simulink model "PMSM_FOC_DualPlant_ClosedLoop_v21"  (R2024a)
settings: Solver=FixedStepDiscrete  StartTime=0.0  StopTime=2.0  FixedStep=0.0001  RelTol=1e-3
model workspace (MAT data in the model file):
  FOC_Native_CurrentIntegratorLimit = Simulink.Parameter
  FOC_Native_CurrentIntegratorLimit.Value = 30
  FOC_Native_CurrentIntegratorLimit.Complexity = 'real'
  FOC_Native_CurrentIntegratorLimit.Dimensions = [1 1]
  FOC_Native_CurrentIntegratorLimit.DataType = 'single'
  FOC_Native_CurrentPeriod = Simulink.Parameter
  FOC_Native_CurrentPeriod.Value = 9.99999974738e-05
  FOC_Native_CurrentPeriod.Complexity = 'real'
  FOC_Native_CurrentPeriod.Dimensions = [1 1]
  FOC_Native_CurrentPeriod.DataType = 'single'
  FOC_Native_DutyMax = Simulink.Parameter
  FOC_Native_DutyMax.Value = 0.980000019073
  FOC_Native_DutyMax.Complexity = 'real'
  FOC_Native_DutyMax.Dimensions = [1 1]
  FOC_Native_DutyMax.DataType = 'single'
  FOC_Native_DutyMin = Simulink.Parameter
  FOC_Native_DutyMin.Value = 0.019999999553
  FOC_Native_DutyMin.Complexity = 'real'
  FOC_Native_DutyMin.Dimensions = [1 1]
  FOC_Native_DutyMin.DataType = 'single'
  FOC_Native_FluxPM = Simulink.Parameter
  FOC_Native_FluxPM.Value = 0.0500000007451
  FOC_Native_FluxPM.Complexity = 'real'
  FOC_Native_FluxPM.Dimensions = [1 1]
  FOC_Native_FluxPM.DataType = 'single'
  FOC_Native_IqLimit = Simulink.Parameter
  FOC_Native_IqLimit.Value = 8
  FOC_Native_IqLimit.Complexity = 'real'
  FOC_Native_IqLimit.Dimensions = [1 1]
  FOC_Native_IqLimit.DataType = 'single'
  FOC_Native_KiCurrent = Simulink.Parameter
  FOC_Native_KiCurrent.Value = 500
  FOC_Native_KiCurrent.Complexity = 'real'
  FOC_Native_KiCurrent.Dimensions = [1 1]
  FOC_Native_KiCurrent.DataType = 'single'
  FOC_Native_KiSpeed = Simulink.Parameter
  FOC_Native_KiSpeed.Value = 0.0500000007451
  FOC_Native_KiSpeed.Complexity = 'real'
  FOC_Native_KiSpeed.Dimensions = [1 1]
  FOC_Native_KiSpeed.DataType = 'single'
  FOC_Native_KpCurrent = Simulink.Parameter
  FOC_Native_KpCurrent.Value = 1
  FOC_Native_KpCurrent.Complexity = 'real'
  FOC_Native_KpCurrent.Dimensions = [1 1]
  FOC_Native_KpCurrent.DataType = 'single'
  FOC_Native_KpSpeed = Simulink.Parameter
  FOC_Native_KpSpeed.Value = 0.019999999553
  FOC_Native_KpSpeed.Complexity = 'real'
  FOC_Native_KpSpeed.Dimensions = [1 1]
  FOC_Native_KpSpeed.DataType = 'single'
  FOC_Native_Ld = Simulink.Parameter
  FOC_Native_Ld.Value = 0.0010000000475
  FOC_Native_Ld.Complexity = 'real'
  FOC_Native_Ld.Dimensions = [1 1]
  FOC_Native_Ld.DataType = 'single'
  FOC_Native_Lq = Simulink.Parameter
  FOC_Native_Lq.Value = 0.0010000000475
  FOC_Native_Lq.Complexity = 'real'
  FOC_Native_Lq.Dimensions = [1 1]
  FOC_Native_Lq.DataType = 'single'
  FOC_Native_PolePairs = Simulink.Parameter
  FOC_Native_PolePairs.Value = 4
  FOC_Native_PolePairs.Complexity = 'real'
  FOC_Native_PolePairs.Dimensions = [1 1]
  FOC_Native_PolePairs.DataType = 'single'
  FOC_Native_SpeedPeriod = Simulink.Parameter
  FOC_Native_SpeedPeriod.Value = 0.0010000000475
  FOC_Native_SpeedPeriod.Complexity = 'real'
  FOC_Native_SpeedPeriod.Dimensions = [1 1]
  FOC_Native_SpeedPeriod.DataType = 'single'
  FOC_Native_VoltageLimit = Simulink.Parameter
  FOC_Native_VoltageLimit.Value = 26
  FOC_Native_VoltageLimit.Complexity = 'real'
  FOC_Native_VoltageLimit.Dimensions = [1 1]
  FOC_Native_VoltageLimit.DataType = 'single'
  NATIVE_INV_SQRT3 = 0.577350258827
  NATIVE_RAD_S_TO_RPM = 9.54929637909
  NATIVE_RPM_TO_RAD_S = 0.104719758034
  NATIVE_SQRT3_BY2 = 0.866025388241
  PMSM_Native_B = 9.99999974738e-05
  PMSM_Native_J = 0.00200000009499
  PMSM_Native_Rs = 0.40000000596
  PMSM_PLANT_SELECTION = 2
values from neighbouring files (symbols this model uses):
  FOC_Native_CurrentIntegratorLimit = 30.0    [PMSM_FOC_Data.sldd]
  FOC_Native_CurrentPeriod = 0.0001    [PMSM_FOC_Data.sldd]
  FOC_Native_DutyMax = 0.98    [PMSM_FOC_Data.sldd]
  FOC_Native_DutyMin = 0.02    [PMSM_FOC_Data.sldd]
  FOC_Native_FluxPM = 0.05    [PMSM_FOC_Data.sldd]
  FOC_Native_IqLimit = 8.0    [PMSM_FOC_Data.sldd]
  FOC_Native_KiCurrent = 500.0    [PMSM_FOC_Data.sldd]
  FOC_Native_KiSpeed = 0.05    [PMSM_FOC_Data.sldd]
  FOC_Native_KpCurrent = 1.0    [PMSM_FOC_Data.sldd]
  FOC_Native_KpSpeed = 0.02    [PMSM_FOC_Data.sldd]
  FOC_Native_Ld = 0.001    [PMSM_FOC_Data.sldd]
  FOC_Native_Lq = 0.001    [PMSM_FOC_Data.sldd]
  FOC_Native_PolePairs = 4.0    [PMSM_FOC_Data.sldd]
  FOC_Native_SpeedPeriod = 0.001    [PMSM_FOC_Data.sldd]
  FOC_Native_VoltageLimit = 26.0    [PMSM_FOC_Data.sldd]
libraries: mcbhdlplantlib x2
settings Model: Creator=18283  LastModifiedBy=18283
settings DataIOCC: SignalLogging=off

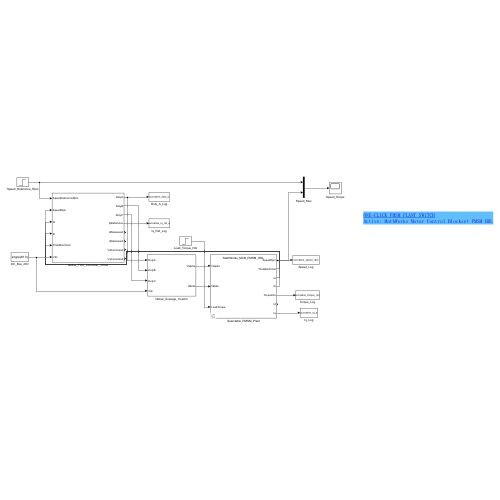
[thumbnail: Simulink's stored preview of the top-level diagram]
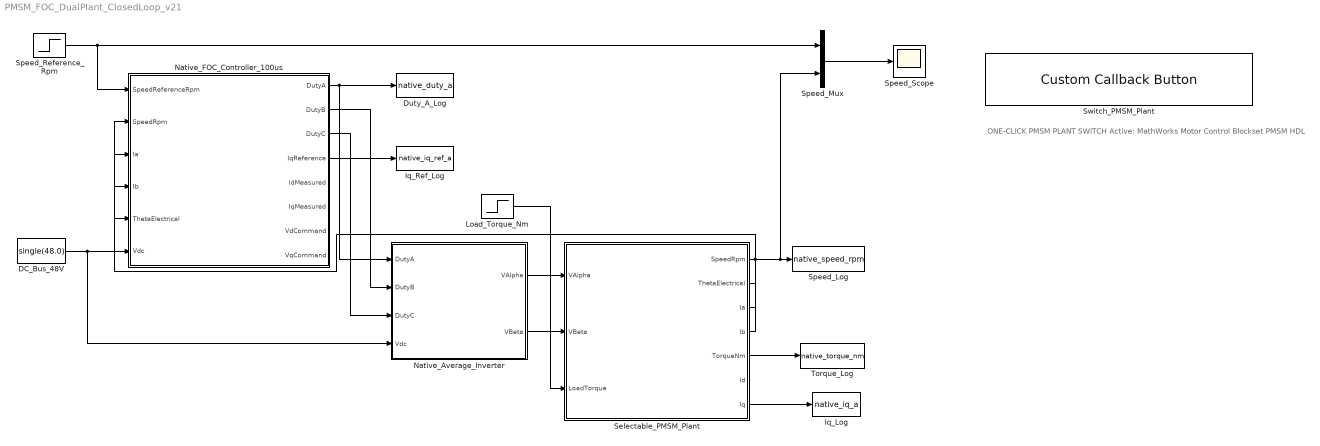
== system PMSM_FOC_DualPlant_ClosedLoop_v21 ==
  note: ONE-CLICK PMSM PLANT SWITCH
      | Active: MathWorks Motor Control Blockset PMSM HDL
  DC_Bus_48V : Constant  Value=single(48.0)  OutDataTypeStr=single
  Duty_A_Log : ToWorkspace  VariableName=native_duty_a  SaveFormat=Timeseries  SampleTime=-1
      settings: MaxDataPoints=20000
  Iq_Log : ToWorkspace  VariableName=native_iq_a  SaveFormat=Timeseries  SampleTime=-1
      settings: MaxDataPoints=20000
  Iq_Ref_Log : ToWorkspace  VariableName=native_iq_ref_a  SaveFormat=Timeseries  SampleTime=-1
      settings: MaxDataPoints=20000
  Load_Torque_Nm : Step  Time=0.5  After=0.2  OutDataTypeStr=single  SampleTime=0.0001
  Native_Average_Inverter : Subsystem
  Native_FOC_Controller_100us : Subsystem
  Selectable_PMSM_Plant : Subsystem  Variant=on  VariantControl=Native_Discrete_PMSM_Plant
  Speed_Log : ToWorkspace  VariableName=native_speed_rpm  SaveFormat=Timeseries  SampleTime=-1
      settings: MaxDataPoints=20000
  Speed_Mux : Mux  Inputs=2
  Speed_Reference_Rpm : Step  Time=0.05  After=1000  OutDataTypeStr=single  SampleTime=0.0001
  Speed_Scope : Scope
  Switch_PMSM_Plant : CustomCallbackButton  Configuration="{\"components\":[{\"name\":\"BackgroundImageComponent\",\"settings\":{\"image\":{\"size\":[0,0],\"src\":\"default\",\"srcOrientation\":\"Right\"},\"position\":[0,0,1,1]}},{\"name\":\"ButtonStateComponent\",\"settings\":{\"buttonType\":\"momentary\",\"clickFcn\":\"run(fullfile('G:\\\\Data\\\\GitFiles\\\\MatlabProgram\\\\Matlab_Projects\\\\PMSM_FOC\\\\model_codegen\\\\PMSM_FOC_DualPlant_v2.1.0','switch_pmsm_plant_v21.m'))\",\"onValue\":1,\"position\":[0,0,1,1],\"pressDelay\":\"500\",\"pressFcn\":\"\",\"repeatInterval\":\"0\",\"states\":[{\"horizontalAlignment\":\"center\",\"image\":{\"position\":[0,0,1,1],\"src\":\"default\",\"srcOrientation\":\"Right\"},\"label\":{\"color\":[0.01176470588,0.01176470588,0.01176470588,1],\"icon\":{\"size\":[0,0],\"src\":\"default\",\"srcOrientation\":\"Right\"},\"iconPlacement\":\"left\",\"text\":{\"content\":\"Active: MathWorks MCB PMSM HDL (click to switch)\"}},\"labelOffset\":[0,0],\"verticalAlignment\":\"middle\"},{\"horizontalAlignment\":\"center\",\"image\":{\"position\":[0,0,1,1],\"src\":\"default\",\"srcOrientation\":\"Right\"},\"label\":{\"color\":[0.01176470588,0.01176470588,0.01176470588,1],\"icon\":{\"size\":[0,0],\"src\":\"default\",\"srcOrientation\":\"Right\"},\"iconPlacement\":\"left\",\"text\":{\"content\":\"Active: MathWorks MCB PMSM HDL (click to switch)\"}},\"labelOffset\":[0,0],\"verticalAlignment\":\"middle\"},{\"horizontalAlignment\":\"center\",\"image\":{\"position\":[0,0,1,1],\"src\":\"default\",\"srcOrientation\":\"Right\"},\"label\":{\"color\":[0.01176470588,0.01176470588,0.01176470588,1],\"icon\":{\"size\":[0,0],\"src\":\"default\",\"srcOrientation\":\"Right\"},\"iconPlacement\":\"left\",\"text\":{\"content\":\"Active: MathWorks MCB PMSM HDL (click to switch)\"}},\"labelOffset\":[0,0],\"verticalAlignment\":\"middle\"},{\"horizontalAlignment\":\"center\",\"image\":{\"position\":[0,0,1,1],\"src\":\"default\",\"srcOrientation\":\"Right\"},\"label\":{\"color\":[0.01176470588,0.01176470588,0.01176470588,1],\"icon\":{\"size\":[0,0],\"src\":\"default\",\"srcOrientation\":\"Right\"},\"iconPlacement\":\"left\",\"text\":{\"content\":\"Active: MathWorks MCB PMSM HDL (click to switch)\"}},\"labelOffset\":[0,0],\"verticalAlignment\":\"middle\"}]}},{\"name\":\"ForegroundImageComponent\",\"settings\":{\"image\":{\"size\":[0,0],\"src\":\"default\",\"srcOrientation\":\"Right\"},\"isForeground\":1,\"position\":[0,0,1,1]}}],\"settings\":{\"BindingType\":\"standalone\",\"backgroundColor\":[244,244,244,1],\"backgroundOffset\":0.2,\"backgroundOpacity\":1,\"fixedAspectRatio\":\"off\",\"foregroundColor\":[0.01176470588,0.01176470588,0.01176470588,1],\"migratedFromLegacy\":true,\"useBackgroundColor\":true,\"variant\":\"callback\",\"version\":\"R2023a\"},\"type\":\"Button\"}"  CustomBackgroundColor="{\"color\":[0.9568627451,0.9568627451,0.9568627451],\"show\":true}"
  Torque_Log : ToWorkspace  VariableName=native_torque_nm  SaveFormat=Timeseries  SampleTime=-1
      settings: MaxDataPoints=20000
  wires:
  Native_FOC_Controller_100us/1(DutyA) -> Native_Average_Inverter/1(DutyA), Duty_A_Log/1
  Speed_Reference_Rpm/1 -> Speed_Mux/1, Native_FOC_Controller_100us/1(SpeedReferenceRpm)
  DC_Bus_48V/1 -> Native_Average_Inverter/4(Vdc), Native_FOC_Controller_100us/6(Vdc)
  Native_FOC_Controller_100us/2(DutyB) -> Native_Average_Inverter/2(DutyB)
  Native_FOC_Controller_100us/3(DutyC) -> Native_Average_Inverter/3(DutyC)
  Native_FOC_Controller_100us/4(IqReference) -> Iq_Ref_Log/1
  Speed_Mux/1 -> Speed_Scope/1
  Native_Average_Inverter/1(VAlpha) -> Selectable_PMSM_Plant/1(VAlpha)
  Native_Average_Inverter/2(VBeta) -> Selectable_PMSM_Plant/2(VBeta)
  Load_Torque_Nm/1 -> Selectable_PMSM_Plant/3(LoadTorque)
  Selectable_PMSM_Plant/1(SpeedRpm) -> Speed_Mux/2, Speed_Log/1, Native_FOC_Controller_100us/2(SpeedRpm)
  Selectable_PMSM_Plant/2(ThetaElectrical) -> Native_FOC_Controller_100us/5(ThetaElectrical)
  Selectable_PMSM_Plant/3(Ia) -> Native_FOC_Controller_100us/3(Ia)
  Selectable_PMSM_Plant/4(Ib) -> Native_FOC_Controller_100us/4(Ib)
  Selectable_PMSM_Plant/5(TorqueNm) -> Torque_Log/1
  Selectable_PMSM_Plant/7(Iq) -> Iq_Log/1

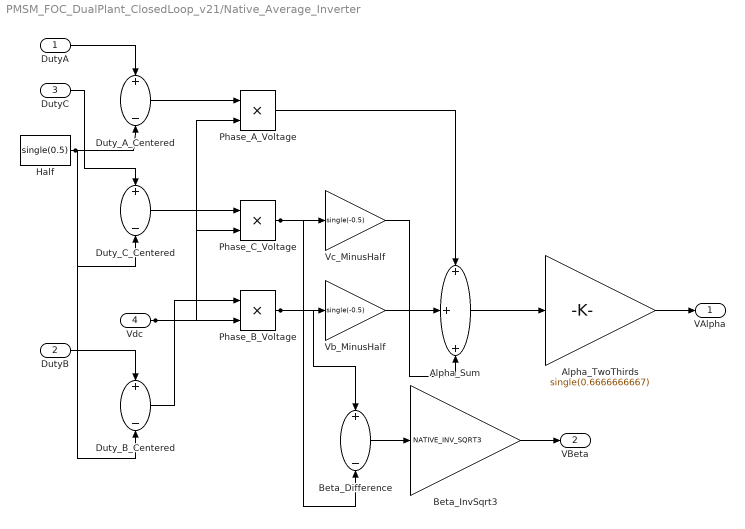
== system PMSM_FOC_DualPlant_ClosedLoop_v21/Native_Average_Inverter ==
  DutyA : Inport  OutDataTypeStr=single
  DutyB : Inport  Port=2  OutDataTypeStr=single
  DutyC : Inport  Port=3  OutDataTypeStr=single
  Vdc : Inport  Port=4  OutDataTypeStr=single
  Alpha_Sum : Sum  Inputs=+++
  Alpha_TwoThirds : Gain  Gain=single(0.6666666667)
  Beta_Difference : Sum  Inputs=+-
  Beta_InvSqrt3 : Gain  Gain=NATIVE_INV_SQRT3
  Duty_A_Centered : Sum  Inputs=+-
  Duty_B_Centered : Sum  Inputs=+-
  Duty_C_Centered : Sum  Inputs=+-
  Half : Constant  Value=single(0.5)  OutDataTypeStr=single
  Phase_A_Voltage : Product  Inputs=**
  Phase_B_Voltage : Product  Inputs=**
  Phase_C_Voltage : Product  Inputs=**
  Vb_MinusHalf : Gain  Gain=single(-0.5)
  Vc_MinusHalf : Gain  Gain=single(-0.5)
  VAlpha : Outport  OutDataTypeStr=single
  VBeta : Outport  Port=2  OutDataTypeStr=single
  wires:
  Beta_Difference/1 -> Beta_InvSqrt3/1
  Duty_B_Centered/1 -> Phase_B_Voltage/1
  Vdc/1 -> Phase_A_Voltage/2, Phase_B_Voltage/2, Phase_C_Voltage/2
  Half/1 -> Duty_C_Centered/2, Duty_B_Centered/2, Duty_A_Centered/2
  DutyA/1 -> Duty_A_Centered/1
  DutyC/1 -> Duty_C_Centered/1
  DutyB/1 -> Duty_B_Centered/1
  Duty_A_Centered/1 -> Phase_A_Voltage/1
  Duty_C_Centered/1 -> Phase_C_Voltage/1
  Phase_A_Voltage/1 -> Alpha_Sum/1
  Phase_C_Voltage/1 -> Beta_Difference/2, Vc_MinusHalf/1
  Phase_B_Voltage/1 -> Beta_Difference/1, Vb_MinusHalf/1
  Vc_MinusHalf/1 -> Alpha_Sum/3
  Vb_MinusHalf/1 -> Alpha_Sum/2
  Alpha_Sum/1 -> Alpha_TwoThirds/1
  Beta_InvSqrt3/1 -> VBeta/1
  Alpha_TwoThirds/1 -> VAlpha/1

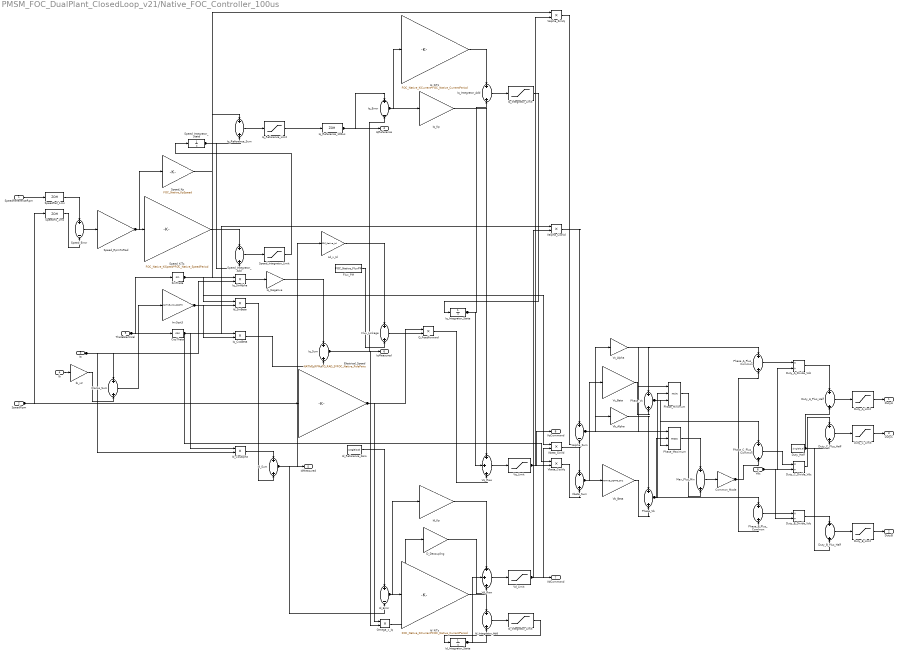
== system PMSM_FOC_DualPlant_ClosedLoop_v21/Native_FOC_Controller_100us ==
  SpeedReferenceRpm : Inport  OutDataTypeStr=single
  SpeedRpm : Inport  Port=2  OutDataTypeStr=single
  Ia : Inport  Port=3  OutDataTypeStr=single
  Ib : Inport  Port=4  OutDataTypeStr=single
  ThetaElectrical : Inport  Port=5  OutDataTypeStr=single
  Vdc : Inport  Port=6  OutDataTypeStr=single
  Clarke_Sum : Sum
  Common_Mode : Gain  Gain=single(-0.5)
  CosTheta : Trigonometry  Operator=cos
  D_Decoupling : Gain  Gain=-FOC_Native_Lq
  Duty_A_Divide_Vdc : Product  Inputs=*/
  Duty_A_Limit : Saturate  UpperLimit=FOC_Native_DutyMax  LowerLimit=FOC_Native_DutyMin
  Duty_A_Plus_Half : Sum
  Duty_B_Divide_Vdc : Product  Inputs=*/
  Duty_B_Limit : Saturate  UpperLimit=FOC_Native_DutyMax  LowerLimit=FOC_Native_DutyMin
  Duty_B_Plus_Half : Sum
  Duty_C_Divide_Vdc : Product  Inputs=*/
  Duty_C_Limit : Saturate  UpperLimit=FOC_Native_DutyMax  LowerLimit=FOC_Native_DutyMin
  Duty_C_Plus_Half : Sum
  Duty_Half : Constant  Value=single(0.5)  OutDataTypeStr=single
  Electrical_Speed : Gain  Gain=NATIVE_RPM_TO_RAD_S*FOC_Native_PolePairs
  Flux_Linkage : Sum
  Flux_PM : Constant  Value=FOC_Native_FluxPM  OutDataTypeStr=single
  Ib_x2 : Gain  Gain=single(2.0)
  Id_CosAlpha : Product  Inputs=**
  Id_Error : Sum  Inputs=+-
  Id_Integrator_Add : Sum
  Id_Integrator_Limit : Saturate  UpperLimit=FOC_Native_CurrentIntegratorLimit  LowerLimit=-FOC_Native_CurrentIntegratorLimit
  Id_Integrator_State : UnitDelay  InitialCondition=single(0.0)  SampleTime=0.0001  HasFrameUpgradeWarning=on
  Id_KiTs : Gain  Gain=FOC_Native_KiCurrent*FOC_Native_CurrentPeriod
  Id_Kp : Gain  Gain=FOC_Native_KpCurrent
  Id_Reference_Zero : Constant  Value=single(0.0)  OutDataTypeStr=single
  Id_SinBeta : Product  Inputs=**
  Id_Sum : Sum
  InvSqrt3 : Gain  Gain=NATIVE_INV_SQRT3
  Iq_CosBeta : Product  Inputs=**
  Iq_Error : Sum  Inputs=+-
  Iq_Integrator_Add : Sum
  Iq_Integrator_Limit : Saturate  UpperLimit=FOC_Native_CurrentIntegratorLimit  LowerLimit=-FOC_Native_CurrentIntegratorLimit
  Iq_Integrator_State : UnitDelay  InitialCondition=single(0.0)  SampleTime=0.0001  HasFrameUpgradeWarning=on
  Iq_KiTs : Gain  Gain=FOC_Native_KiCurrent*FOC_Native_CurrentPeriod
  Iq_Kp : Gain  Gain=FOC_Native_KpCurrent
  Iq_Negative : Gain  Gain=single(-1.0)
  Iq_Reference_100us : ZeroOrderHold  SampleTime=0.0001
  Iq_Reference_Limit : Saturate  UpperLimit=FOC_Native_IqLimit  LowerLimit=-FOC_Native_IqLimit
  Iq_Reference_Sum : Sum
  Iq_SinAlpha : Product  Inputs=**
  Iq_Sum : Sum
  Ld_x_Id : Gain  Gain=FOC_Native_Ld
  Max_Plus_Min : Sum
  Omega_x_Iq : Product  Inputs=**
  Phase_A_Plus_Common : Sum
  Phase_B_Plus_Common : Sum
  Phase_C_Plus_Common : Sum
  Phase_Maximum : MinMax  Function=max  Inputs=3
  Phase_Minimum : MinMax  Inputs=3
  Phase_Vb : Sum
  Phase_Vc : Sum
  Q_Feedforward : Product  Inputs=**
  SinTheta : Trigonometry
  SpeedFb_1ms : ZeroOrderHold  SampleTime=0.001
  SpeedRef_1ms : ZeroOrderHold  SampleTime=0.001
  Speed_Error : Sum  Inputs=+-
  Speed_Integrator_Add : Sum
  Speed_Integrator_Limit : Saturate  UpperLimit=FOC_Native_IqLimit  LowerLimit=-FOC_Native_IqLimit
  Speed_Integrator_State : UnitDelay  InitialCondition=single(0.0)  SampleTime=0.001  HasFrameUpgradeWarning=on
  Speed_KiTs : Gain  Gain=FOC_Native_KiSpeed*FOC_Native_SpeedPeriod
  Speed_Kp : Gain  Gain=FOC_Native_KpSpeed
  Speed_RpmToRad : Gain  Gain=NATIVE_RPM_TO_RAD_S
  Valpha_CosVd : Product  Inputs=**
  Valpha_SinVq : Product  Inputs=**
  Valpha_Sum : Sum  Inputs=+-
  Vb_Alpha : Gain  Gain=single(-0.5)
  Vb_Beta : Gain  Gain=NATIVE_SQRT3_BY2
  Vbeta_CosVq : Product  Inputs=**
  Vbeta_SinVd : Product  Inputs=**
  Vbeta_Sum : Sum
  Vc_Alpha : Gain  Gain=single(-0.5)
  Vc_Beta : Gain  Gain=-NATIVE_SQRT3_BY2
  Vd_Limit : Saturate  UpperLimit=FOC_Native_VoltageLimit  LowerLimit=-FOC_Native_VoltageLimit
  Vd_Raw : Sum  Inputs=+++
  Vq_Limit : Saturate  UpperLimit=FOC_Native_VoltageLimit  LowerLimit=-FOC_Native_VoltageLimit
  Vq_Raw : Sum  Inputs=+++
  DutyA : Outport  OutDataTypeStr=single
  DutyB : Outport  Port=2  OutDataTypeStr=single
  DutyC : Outport  Port=3  OutDataTypeStr=single
  IqReference : Outport  Port=4  OutDataTypeStr=single
  IdMeasured : Outport  Port=5  OutDataTypeStr=single
  IqMeasured : Outport  Port=6  OutDataTypeStr=single
  VdCommand : Outport  Port=7  OutDataTypeStr=single
  VqCommand : Outport  Port=8  OutDataTypeStr=single
  wires:
  SpeedReferenceRpm/1 -> SpeedRef_1ms/1
  Clarke_Sum/1 -> InvSqrt3/1
  Phase_Vb/1 -> Phase_Maximum/2, Phase_B_Plus_Common/1, Phase_Minimum/2
  Speed_Error/1 -> Speed_RpmToRad/1
  Max_Plus_Min/1 -> Common_Mode/1
  Id_Integrator_Add/1 -> Id_Integrator_Limit/1
  SpeedRpm/1 -> Electrical_Speed/1, SpeedFb_1ms/1
  CosTheta/1 -> Vbeta_CosVq/1, Valpha_CosVd/1, Iq_CosBeta/1, Id_CosAlpha/1
  Ia/1 -> Clarke_Sum/1, Id_CosAlpha/2, Iq_SinAlpha/2
  SpeedRef_1ms/1 -> Speed_Error/1
  Vb_Beta/1 -> Phase_Vb/2
  Duty_B_Divide_Vdc/1 -> Duty_B_Plus_Half/1
  D_Decoupling/1 -> Vd_Raw/3
  Ib_x2/1 -> Clarke_Sum/2
  Duty_A_Limit/1 -> DutyA/1
  Iq_Integrator_Add/1 -> Iq_Integrator_Limit/1
  Ib/1 -> Ib_x2/1
  SpeedFb_1ms/1 -> Speed_Error/2
  Speed_RpmToRad/1 -> Speed_KiTs/1, Speed_Kp/1
  Flux_Linkage/1 -> Q_Feedforward/2
  Iq_Reference_Limit/1 -> Iq_Reference_100us/1
  Omega_x_Iq/1 -> D_Decoupling/1
  ThetaElectrical/1 -> SinTheta/1, CosTheta/1
  Speed_Integrator_State/1 -> Iq_Reference_Sum/2, Speed_Integrator_Add/2
  Speed_Kp/1 -> Iq_Reference_Sum/1
  Speed_KiTs/1 -> Speed_Integrator_Add/1
  Id_KiTs/1 -> Id_Integrator_Add/1
  Phase_Vc/1 -> Phase_Maximum/3, Phase_C_Plus_Common/1, Phase_Minimum/3
  SinTheta/1 -> Vbeta_SinVd/1, Iq_SinAlpha/1, Id_SinBeta/1, Valpha_SinVq/1
  Id_Kp/1 -> Vd_Raw/1
  InvSqrt3/1 -> Id_SinBeta/2, Iq_CosBeta/2
  Iq_Reference_Sum/1 -> Iq_Reference_Limit/1
  Speed_Integrator_Add/1 -> Speed_Integrator_Limit/1
  Valpha_Sum/1 -> Phase_Maximum/1, Phase_Minimum/1, Phase_A_Plus_Common/1, Vc_Alpha/1, Vb_Alpha/1
  Common_Mode/1 -> Phase_C_Plus_Common/2, Phase_B_Plus_Common/2, Phase_A_Plus_Common/2
  Iq_SinAlpha/1 -> Iq_Negative/1
  Valpha_CosVd/1 -> Valpha_Sum/1
  Id_SinBeta/1 -> Id_Sum/2
  Iq_CosBeta/1 -> Iq_Sum/2
  Id_CosAlpha/1 -> Id_Sum/1
  Valpha_SinVq/1 -> Valpha_Sum/2
  Id_Integrator_State/1 -> Id_Integrator_Add/2, Vd_Raw/2
  Phase_Minimum/1 -> Max_Plus_Min/2
  Speed_Integrator_Limit/1 -> Speed_Integrator_State/1
  Iq_Negative/1 -> Iq_Sum/1
  Id_Sum/1 -> IdMeasured/1, Id_Error/2, Ld_x_Id/1
  Iq_Reference_100us/1 -> Iq_Error/1, IqReference/1
  Ld_x_Id/1 -> Flux_Linkage/1
  Flux_PM/1 -> Flux_Linkage/2
  Vd_Limit/1 -> Valpha_CosVd/2, Vbeta_SinVd/2, VdCommand/1
  Iq_Sum/1 -> Iq_Error/2, IqMeasured/1, Omega_x_Iq/2
  Electrical_Speed/1 -> Q_Feedforward/1, Omega_x_Iq/1
  Id_Reference_Zero/1 -> Id_Error/1
  Vq_Raw/1 -> Vq_Limit/1
  Iq_Error/1 -> Iq_KiTs/1, Iq_Kp/1
  Id_Error/1 -> Id_Kp/1, Id_KiTs/1
  Iq_KiTs/1 -> Iq_Integrator_Add/1
  Iq_Kp/1 -> Vq_Raw/1
  Iq_Integrator_State/1 -> Vq_Raw/2, Iq_Integrator_Add/2
  Q_Feedforward/1 -> Vq_Raw/3
  Vc_Alpha/1 -> Phase_Vc/1
  Vd_Raw/1 -> Vd_Limit/1
  Vc_Beta/1 -> Phase_Vc/2
  Iq_Integrator_Limit/1 -> Iq_Integrator_State/1
  Vq_Limit/1 -> Valpha_SinVq/2, VqCommand/1, Vbeta_CosVq/2
  Vb_Alpha/1 -> Phase_Vb/1
  Id_Integrator_Limit/1 -> Id_Integrator_State/1
  Vbeta_SinVd/1 -> Vbeta_Sum/1
  Vbeta_CosVq/1 -> Vbeta_Sum/2
  Vbeta_Sum/1 -> Vb_Beta/1, Vc_Beta/1
  Phase_Maximum/1 -> Max_Plus_Min/1
  Phase_A_Plus_Common/1 -> Duty_A_Divide_Vdc/1
  Phase_C_Plus_Common/1 -> Duty_C_Divide_Vdc/1
  Vdc/1 -> Duty_A_Divide_Vdc/2, Duty_B_Divide_Vdc/2, Duty_C_Divide_Vdc/2
  Phase_B_Plus_Common/1 -> Duty_B_Divide_Vdc/1
  Duty_A_Divide_Vdc/1 -> Duty_A_Plus_Half/1
  Duty_Half/1 -> Duty_B_Plus_Half/2, Duty_A_Plus_Half/2, Duty_C_Plus_Half/2
  Duty_C_Divide_Vdc/1 -> Duty_C_Plus_Half/1
  Duty_A_Plus_Half/1 -> Duty_A_Limit/1
  Duty_C_Plus_Half/1 -> Duty_C_Limit/1
  Duty_B_Plus_Half/1 -> Duty_B_Limit/1
  Duty_C_Limit/1 -> DutyC/1
  Duty_B_Limit/1 -> DutyB/1

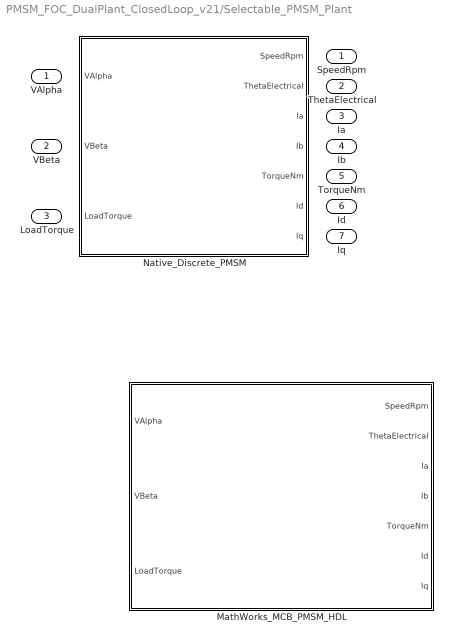
== system PMSM_FOC_DualPlant_ClosedLoop_v21/Selectable_PMSM_Plant ==
  VAlpha : Inport
  VBeta : Inport  Port=2
  LoadTorque : Inport  Port=3
  MathWorks_MCB_PMSM_HDL : Subsystem  VariantControl=PMSM_PLANT_SELECTION == 2
  Native_Discrete_PMSM : Subsystem  VariantControl=PMSM_PLANT_SELECTION == 1
  SpeedRpm : Outport
  ThetaElectrical : Outport  Port=2
  Ia : Outport  Port=3
  Ib : Outport  Port=4
  TorqueNm : Outport  Port=5
  Id : Outport  Port=6
  Iq : Outport  Port=7

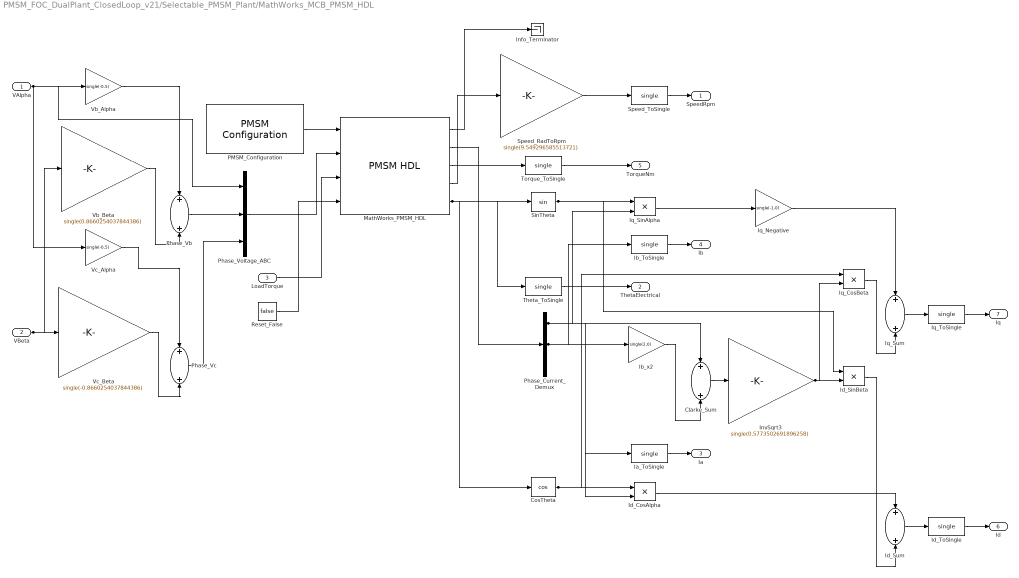
== system PMSM_FOC_DualPlant_ClosedLoop_v21/Selectable_PMSM_Plant/MathWorks_MCB_PMSM_HDL ==
  VAlpha : Inport  OutDataTypeStr=single
  VBeta : Inport  Port=2  OutDataTypeStr=single
  LoadTorque : Inport  Port=3  OutDataTypeStr=single
  Clarke_Sum : Sum
  CosTheta : Trigonometry  Operator=cos
  Ia_ToSingle : DataTypeConversion  OutDataTypeStr=single  SaturateOnIntegerOverflow=off  RndMeth=Floor
  Ib_ToSingle : DataTypeConversion  OutDataTypeStr=single  SaturateOnIntegerOverflow=off  RndMeth=Floor
  Ib_x2 : Gain  Gain=single(2.0)
  Id_CosAlpha : Product  Inputs=**
  Id_SinBeta : Product  Inputs=**
  Id_Sum : Sum
  Id_ToSingle : DataTypeConversion  OutDataTypeStr=single  SaturateOnIntegerOverflow=off  RndMeth=Floor
  Info_Terminator : Terminator
  InvSqrt3 : Gain  Gain=single(0.5773502691896258)
  Iq_CosBeta : Product  Inputs=**
  Iq_Negative : Gain  Gain=single(-1.0)
  Iq_SinAlpha : Product  Inputs=**
  Iq_Sum : Sum
  Iq_ToSingle : DataTypeConversion  OutDataTypeStr=single  SaturateOnIntegerOverflow=off  RndMeth=Floor
  MathWorks_PMSM_HDL : mcbhdlplantlib/PMSM HDL  VariantControl=pmsmVariant==pmsmEnum.TorqueInput  Ts=0.0001
  PMSM_Configuration : mcbhdlplantlib/PMSM Configuration  portConfig=Torque  Trq_N_mode=0  Ts=0.0001  Pp=4  Rs=0.4  Ld=0.001  Lq=0.001  lambda_pm=0.05  J=0.002  B=0.0001  f=0
  Phase_Current_Demux : Demux  Outputs=3
  Phase_Vb : Sum
  Phase_Vc : Sum
  Phase_Voltage_ABC : Mux  Inputs=3
  Reset_False : Constant  Value=false  OutDataTypeStr=boolean
  SinTheta : Trigonometry
  Speed_RadToRpm : Gain  Gain=single(9.549296585513721)
  Speed_ToSingle : DataTypeConversion  OutDataTypeStr=single  SaturateOnIntegerOverflow=off  RndMeth=Floor
  Theta_ToSingle : DataTypeConversion  OutDataTypeStr=single  SaturateOnIntegerOverflow=off  RndMeth=Floor
  Torque_ToSingle : DataTypeConversion  OutDataTypeStr=single  SaturateOnIntegerOverflow=off  RndMeth=Floor
  Vb_Alpha : Gain  Gain=single(-0.5)
  Vb_Beta : Gain  Gain=single(0.8660254037844386)
  Vc_Alpha : Gain  Gain=single(-0.5)
  Vc_Beta : Gain  Gain=single(-0.8660254037844386)
  SpeedRpm : Outport  OutDataTypeStr=single
  ThetaElectrical : Outport  Port=2  OutDataTypeStr=single
  Ia : Outport  Port=3  OutDataTypeStr=single
  Ib : Outport  Port=4  OutDataTypeStr=single
  TorqueNm : Outport  Port=5  OutDataTypeStr=single
  Id : Outport  Port=6  OutDataTypeStr=single
  Iq : Outport  Port=7  OutDataTypeStr=single
  wires:
  Vc_Beta/1 -> Phase_Vc/2
  Id_Sum/1 -> Id_ToSingle/1
  MathWorks_PMSM_HDL/5 -> Theta_ToSingle/1, SinTheta/1, CosTheta/1
  VAlpha/1 -> Vc_Alpha/1, Vb_Alpha/1, Phase_Voltage_ABC/1
  Phase_Vc/1 -> Phase_Voltage_ABC/3
  Iq_SinAlpha/1 -> Iq_Negative/1
  VBeta/1 -> Vb_Beta/1, Vc_Beta/1
  Vb_Alpha/1 -> Phase_Vb/1
  Vb_Beta/1 -> Phase_Vb/2
  Vc_Alpha/1 -> Phase_Vc/1
  Phase_Vb/1 -> Phase_Voltage_ABC/2
  PMSM_Configuration/1 -> MathWorks_PMSM_HDL/1
  Phase_Voltage_ABC/1 -> MathWorks_PMSM_HDL/2
  LoadTorque/1 -> MathWorks_PMSM_HDL/3
  Reset_False/1 -> MathWorks_PMSM_HDL/4
  Id_SinBeta/1 -> Id_Sum/2
  MathWorks_PMSM_HDL/2 -> Phase_Current_Demux/1
  MathWorks_PMSM_HDL/1 -> Info_Terminator/1
  MathWorks_PMSM_HDL/4 -> Speed_RadToRpm/1
  MathWorks_PMSM_HDL/3 -> Torque_ToSingle/1
  Speed_RadToRpm/1 -> Speed_ToSingle/1
  Torque_ToSingle/1 -> TorqueNm/1
  SinTheta/1 -> Id_SinBeta/1, Iq_SinAlpha/1
  Theta_ToSingle/1 -> ThetaElectrical/1
  Phase_Current_Demux/2 -> Ib_ToSingle/1, Ib_x2/1
  Phase_Current_Demux/1 -> Clarke_Sum/1, Id_CosAlpha/2, Iq_SinAlpha/2, Ia_ToSingle/1
  CosTheta/1 -> Iq_CosBeta/1, Id_CosAlpha/1
  Speed_ToSingle/1 -> SpeedRpm/1
  Ib_ToSingle/1 -> Ib/1
  Ib_x2/1 -> Clarke_Sum/2
  Ia_ToSingle/1 -> Ia/1
  Id_CosAlpha/1 -> Id_Sum/1
  Clarke_Sum/1 -> InvSqrt3/1
  Iq_Negative/1 -> Iq_Sum/1
  InvSqrt3/1 -> Id_SinBeta/2, Iq_CosBeta/2
  Iq_CosBeta/1 -> Iq_Sum/2
  Iq_Sum/1 -> Iq_ToSingle/1
  Iq_ToSingle/1 -> Iq/1
  Id_ToSingle/1 -> Id/1

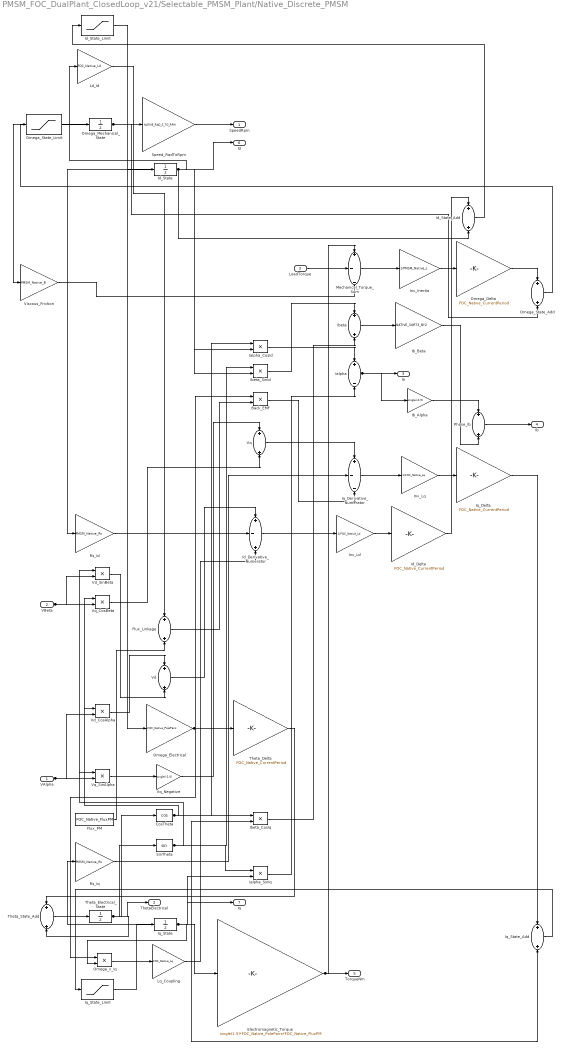
== system PMSM_FOC_DualPlant_ClosedLoop_v21/Selectable_PMSM_Plant/Native_Discrete_PMSM ==
  VAlpha : Inport  OutDataTypeStr=single
  VBeta : Inport  Port=2  OutDataTypeStr=single
  LoadTorque : Inport  Port=3  OutDataTypeStr=single
  Back_EMF : Product  Inputs=**
  CosTheta : Trigonometry  Operator=cos
  Electromagnetic_Torque : Gain  Gain=single(1.5)*FOC_Native_PolePairs*FOC_Native_FluxPM
  Flux_Linkage : Sum
  Flux_PM : Constant  Value=FOC_Native_FluxPM  OutDataTypeStr=single
  Ialpha : Sum  Inputs=+-
  Ialpha_CosId : Product  Inputs=**
  Ialpha_SinIq : Product  Inputs=**
  Ib_Alpha : Gain  Gain=single(-0.5)
  Ib_Beta : Gain  Gain=NATIVE_SQRT3_BY2
  Ibeta : Sum
  Ibeta_CosIq : Product  Inputs=**
  Ibeta_SinId : Product  Inputs=**
  Id_Delta : Gain  Gain=FOC_Native_CurrentPeriod
  Id_Derivative_Numerator : Sum  Inputs=+-+
  Id_State : UnitDelay  InitialCondition=single(0.0)  SampleTime=0.0001  HasFrameUpgradeWarning=on
  Id_State_Add : Sum
  Id_State_Limit : Saturate  UpperLimit=single(20.0)  LowerLimit=single(-20.0)
  Inv_Inertia : Gain  Gain=1/PMSM_Native_J
  Inv_Ld : Gain  Gain=1/FOC_Native_Ld
  Inv_Lq : Gain  Gain=1/FOC_Native_Lq
  Iq_Delta : Gain  Gain=FOC_Native_CurrentPeriod
  Iq_Derivative_Numerator : Sum  Inputs=+--
  Iq_State : UnitDelay  InitialCondition=single(0.0)  SampleTime=0.0001  HasFrameUpgradeWarning=on
  Iq_State_Add : Sum
  Iq_State_Limit : Saturate  UpperLimit=single(20.0)  LowerLimit=single(-20.0)
  Ld_Id : Gain  Gain=FOC_Native_Ld
  Lq_Coupling : Gain  Gain=FOC_Native_Lq
  Mechanical_Torque_Sum : Sum  Inputs=+--
  Omega_Delta : Gain  Gain=FOC_Native_CurrentPeriod
  Omega_Electrical : Gain  Gain=FOC_Native_PolePairs
  Omega_Mechanical_State : UnitDelay  InitialCondition=single(0.0)  SampleTime=0.0001  HasFrameUpgradeWarning=on
  Omega_State_Add : Sum
  Omega_State_Limit : Saturate  UpperLimit=single(500.0)  LowerLimit=single(-500.0)
  Omega_x_Iq : Product  Inputs=**
  Phase_Ib : Sum
  Rs_Id : Gain  Gain=PMSM_Native_Rs
  Rs_Iq : Gain  Gain=PMSM_Native_Rs
  SinTheta : Trigonometry
  Speed_RadToRpm : Gain  Gain=NATIVE_RAD_S_TO_RPM
  Theta_Delta : Gain  Gain=FOC_Native_CurrentPeriod
  Theta_Electrical_State : UnitDelay  InitialCondition=single(0.0)  SampleTime=0.0001  HasFrameUpgradeWarning=on
  Theta_State_Add : Sum
  Vd : Sum
  Vd_CosAlpha : Product  Inputs=**
  Vd_SinBeta : Product  Inputs=**
  Viscous_Friction : Gain  Gain=PMSM_Native_B
  Vq : Sum
  Vq_CosBeta : Product  Inputs=**
  Vq_Negative : Gain  Gain=single(-1.0)
  Vq_SinAlpha : Product  Inputs=**
  SpeedRpm : Outport  OutDataTypeStr=single
  ThetaElectrical : Outport  Port=2  OutDataTypeStr=single
  Ia : Outport  Port=3  OutDataTypeStr=single
  Ib : Outport  Port=4  OutDataTypeStr=single
  TorqueNm : Outport  Port=5  OutDataTypeStr=single
  Id : Outport  Port=6  OutDataTypeStr=single
  Iq : Outport  Port=7  OutDataTypeStr=single
  wires:
  VBeta/1 -> Vd_SinBeta/2, Vq_CosBeta/2
  Omega_State_Limit/1 -> Omega_Mechanical_State/1
  Theta_Delta/1 -> Theta_State_Add/1
  Id_State_Limit/1 -> Id_State/1
  Viscous_Friction/1 -> Mechanical_Torque_Sum/3
  Ibeta_SinId/1 -> Ibeta/1
  VAlpha/1 -> Vd_CosAlpha/2, Vq_SinAlpha/2
  Iq_Derivative_Numerator/1 -> Inv_Lq/1
  Omega_Mechanical_State/1 -> Omega_Electrical/1, Speed_RadToRpm/1, Omega_State_Add/2, Viscous_Friction/1
  Theta_State_Add/1 -> Theta_Electrical_State/1
  Ld_Id/1 -> Flux_Linkage/1
  Rs_Id/1 -> Id_Derivative_Numerator/2
  Phase_Ib/1 -> Ib/1
  Omega_x_Iq/1 -> Lq_Coupling/1
  Vd_SinBeta/1 -> Vd/2
  Vq_CosBeta/1 -> Vq/2
  Vd_CosAlpha/1 -> Vd/1
  Vq_SinAlpha/1 -> Vq_Negative/1
  Ialpha_CosId/1 -> Ialpha/1
  Flux_PM/1 -> Flux_Linkage/2
  Rs_Iq/1 -> Iq_Derivative_Numerator/2
  Ibeta/1 -> Ib_Beta/1
  Theta_Electrical_State/1 -> Theta_State_Add/2, SinTheta/1, CosTheta/1, ThetaElectrical/1
  Iq_State_Limit/1 -> Iq_State/1
  Id_State_Add/1 -> Id_State_Limit/1
  Speed_RadToRpm/1 -> SpeedRpm/1
  Lq_Coupling/1 -> Id_Derivative_Numerator/3
  Id_State/1 -> Rs_Id/1, Ld_Id/1, Id_State_Add/2, Ialpha_CosId/2, Ibeta_SinId/2, Id/1
  Flux_Linkage/1 -> Back_EMF/2
  Vd/1 -> Id_Derivative_Numerator/1
  Omega_Electrical/1 -> Omega_x_Iq/1, Back_EMF/1, Theta_Delta/1
  Ibeta_CosIq/1 -> Ibeta/2
  Vq_Negative/1 -> Vq/1
  Iq_Delta/1 -> Iq_State_Add/1
  CosTheta/1 -> Vd_CosAlpha/1, Ialpha_CosId/1, Vq_CosBeta/1, Ibeta_CosIq/1
  SinTheta/1 -> Vd_SinBeta/1, Vq_SinAlpha/1, Ialpha_SinIq/1, Ibeta_SinId/1
  Omega_State_Add/1 -> Omega_State_Limit/1
  Iq_State/1 -> Omega_x_Iq/2, Iq_State_Add/2, Electromagnetic_Torque/1, Ialpha_SinIq/2, Ibeta_CosIq/2, Rs_Iq/1, Iq/1
  LoadTorque/1 -> Mechanical_Torque_Sum/2
  Back_EMF/1 -> Iq_Derivative_Numerator/3
  Vq/1 -> Iq_Derivative_Numerator/1
  Ib_Alpha/1 -> Phase_Ib/1
  Id_Derivative_Numerator/1 -> Inv_Ld/1
  Ialpha_SinIq/1 -> Ialpha/2
  Electromagnetic_Torque/1 -> TorqueNm/1, Mechanical_Torque_Sum/1
  Mechanical_Torque_Sum/1 -> Inv_Inertia/1
  Ialpha/1 -> Ib_Alpha/1, Ia/1
  Inv_Ld/1 -> Id_Delta/1
  Inv_Inertia/1 -> Omega_Delta/1
  Ib_Beta/1 -> Phase_Ib/2
  Inv_Lq/1 -> Iq_Delta/1
  Id_Delta/1 -> Id_State_Add/1
  Omega_Delta/1 -> Omega_State_Add/1
  Iq_State_Add/1 -> Iq_State_Limit/1
